simulink library "Encoders_Lib"  (R2023a)
settings: Solver=ode45  StartTime=0.0  StopTime=10.0  RelTol=1e-3  EnableMultiTasking=on
settings Model: Creator=uzivatel  LastModifiedBy=Jozko Mrkvicka
settings SolverCC: AlgebraicLoopSolver=TrustRegion
settings DataIOCC: LimitDataPoints=on  SaveFormat=Array  ReturnWorkspaceOutputs=off
settings OptimizationCC: LifeSpan=inf
settings DebuggingCC: UnderspecifiedInitializationDetection=Classic  MergeDetectMultiDrivingBlocksExec=none  SolverPrmCheckMsg=warning  UnconnectedInputMsg=warning  UnconnectedOutputMsg=warning  UnconnectedLineMsg=warning  StateNameClashWarn=warning  SFUnexpectedBacktrackingDiag=warning  SFNoUnconditionalDefaultTransitionDiag=warning  ArithmeticOperatorsInVariantConditions=warning
settings HardwareCC: ProdBitPerPointer=32  ProdBitPerSizeT=32  ProdBitPerPtrDiffT=32  ProdLargestAtomicFloat=None  ProdIntDivRoundTo=Undefined  ProdEndianess=Unspecified  ProdWordSize=32  ProdHWDeviceType=32-bit Generic
settings ModelReferenceCC: EnableRefExpFcnMdlSchedulingChecks=on  PropagateSignalLabelsOutOfModel=off
settings SFSimCC: SimUseLocalCustomCode=off  CustomCodeUndefinedFunction=UseInterfaceOnly
settings RTWCC: RTWUseLocalCustomCode=off
settings CodeAppCC: StateflowObjectComments=on
settings GRTTargetCC: TargetLangStandard=C89/C90 (ANSI)
settings ConfigComp: CovMetricSettings=dw  CovSaveCumulativeToWorkspaceVar=on  CovSaveSingleToWorkspaceVar=on  CovExternalEMLEnable=off

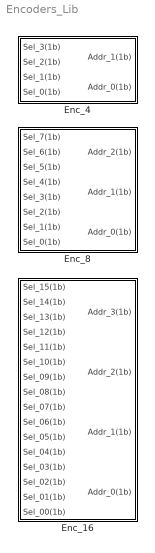
== system Encoders_Lib ==
  Enc_16 : Subsystem
  Enc_4 : Subsystem
  Enc_8 : Subsystem

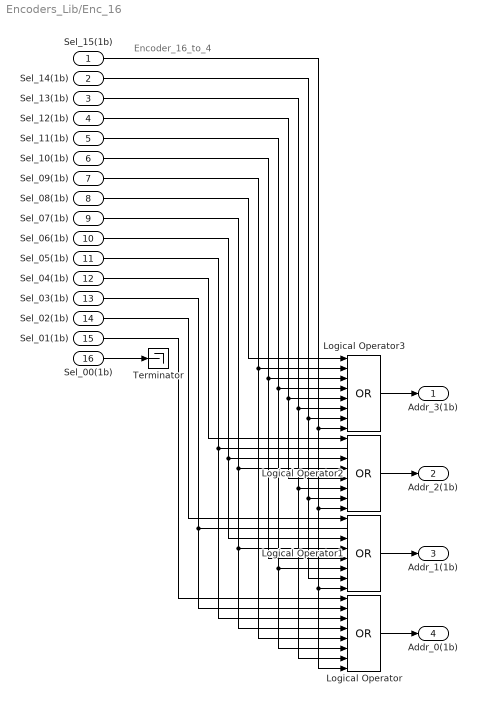
== system Encoders_Lib/Enc_16 ==
  note: Encoder_16_to_4
  Sel_15(1b) : Inport
  Sel_14(1b) : Inport  Port=2
  Sel_13(1b) : Inport  Port=3
  Sel_12(1b) : Inport  Port=4
  Sel_11(1b) : Inport  Port=5
  Sel_10(1b) : Inport  Port=6
  Sel_09(1b) : Inport  Port=7
  Sel_08(1b) : Inport  Port=8
  Sel_07(1b) : Inport  Port=9
  Sel_06(1b) : Inport  Port=10
  Sel_05(1b) : Inport  Port=11
  Sel_04(1b) : Inport  Port=12
  Sel_03(1b) : Inport  Port=13
  Sel_02(1b) : Inport  Port=14
  Sel_01(1b) : Inport  Port=15
  Sel_00(1b) : Inport  Port=16
  Logical Operator{,1..3} (4 alike) : Logic  Operator=OR  Inputs=8  IconShape=distinctive  AllPortsSameDT=off  OutDataTypeStr=boolean
  Terminator : Terminator
  Addr_3(1b) : Outport
  Addr_2(1b) : Outport  Port=2
  Addr_1(1b) : Outport  Port=3
  Addr_0(1b) : Outport  Port=4
  wires:
  Logical Operator/1 -> Addr_0(1b)/1
  Logical Operator1/1 -> Addr_1(1b)/1
  Logical Operator2/1 -> Addr_2(1b)/1
  Logical Operator3/1 -> Addr_3(1b)/1
  Sel_01(1b)/1 -> Logical Operator/1
  Sel_02(1b)/1 -> Logical Operator1/1
  Sel_03(1b)/1 -> Logical Operator1/2, Logical Operator/2
  Sel_04(1b)/1 -> Logical Operator2/1
  Sel_05(1b)/1 -> Logical Operator2/2, Logical Operator/3
  Sel_06(1b)/1 -> Logical Operator2/3, Logical Operator1/3
  Sel_07(1b)/1 -> Logical Operator2/4, Logical Operator/4, Logical Operator1/4
  Sel_08(1b)/1 -> Logical Operator3/1
  Sel_09(1b)/1 -> Logical Operator/5, Logical Operator3/2
  Sel_10(1b)/1 -> Logical Operator1/5, Logical Operator3/3
  Sel_11(1b)/1 -> Logical Operator3/4, Logical Operator/6, Logical Operator1/6
  Sel_12(1b)/1 -> Logical Operator2/5, Logical Operator3/5
  Sel_13(1b)/1 -> Logical Operator/7, Logical Operator2/6, Logical Operator3/6
  Sel_14(1b)/1 -> Logical Operator3/7, Logical Operator1/7, Logical Operator2/7
  Sel_15(1b)/1 -> Logical Operator/8, Logical Operator1/8, Logical Operator2/8, Logical Operator3/8
  Sel_00(1b)/1 -> Terminator/1

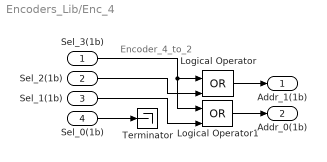
== system Encoders_Lib/Enc_4 ==
  note: Encoder_4_to_2
  Sel_3(1b) : Inport
  Sel_2(1b) : Inport  Port=2
  Sel_1(1b) : Inport  Port=3
  Sel_0(1b) : Inport  Port=4
  Logical Operator : Logic  Operator=OR  IconShape=distinctive  AllPortsSameDT=off  OutDataTypeStr=boolean
  Logical Operator1 : Logic  Operator=OR  IconShape=distinctive  AllPortsSameDT=off  OutDataTypeStr=boolean
  Terminator : Terminator
  Addr_1(1b) : Outport
  Addr_0(1b) : Outport  Port=2
  wires:
  Logical Operator/1 -> Addr_1(1b)/1
  Logical Operator1/1 -> Addr_0(1b)/1
  Sel_2(1b)/1 -> Logical Operator/2
  Sel_1(1b)/1 -> Logical Operator1/2
  Sel_0(1b)/1 -> Terminator/1
  Sel_3(1b)/1 -> Logical Operator/1, Logical Operator1/1

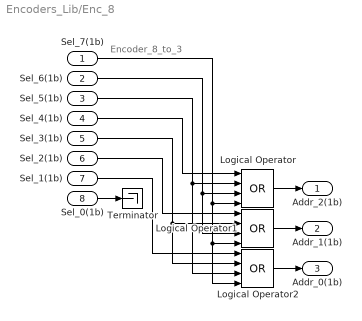
== system Encoders_Lib/Enc_8 ==
  note: Encoder_8_to_3
  Sel_7(1b) : Inport
  Sel_6(1b) : Inport  Port=2
  Sel_5(1b) : Inport  Port=3
  Sel_4(1b) : Inport  Port=4
  Sel_3(1b) : Inport  Port=5
  Sel_2(1b) : Inport  Port=6
  Sel_1(1b) : Inport  Port=7
  Sel_0(1b) : Inport  Port=8
  Logical Operator : Logic  Operator=OR  Inputs=4  IconShape=distinctive  AllPortsSameDT=off  OutDataTypeStr=boolean
  Logical Operator1 : Logic  Operator=OR  Inputs=4  IconShape=distinctive  AllPortsSameDT=off  OutDataTypeStr=boolean
  Logical Operator2 : Logic  Operator=OR  Inputs=4  IconShape=distinctive  AllPortsSameDT=off  OutDataTypeStr=boolean
  Terminator : Terminator
  Addr_2(1b) : Outport
  Addr_1(1b) : Outport  Port=2
  Addr_0(1b) : Outport  Port=3
  wires:
  Logical Operator/1 -> Addr_2(1b)/1
  Logical Operator1/1 -> Addr_1(1b)/1
  Logical Operator2/1 -> Addr_0(1b)/1
  Sel_4(1b)/1 -> Logical Operator/1
  Sel_2(1b)/1 -> Logical Operator1/1
  Sel_6(1b)/1 -> Logical Operator/3, Logical Operator1/3
  Sel_5(1b)/1 -> Logical Operator/2, Logical Operator2/3
  Sel_3(1b)/1 -> Logical Operator2/2, Logical Operator1/2
  Sel_7(1b)/1 -> Logical Operator/4, Logical Operator2/4, Logical Operator1/4
  Sel_0(1b)/1 -> Terminator/1
  Sel_1(1b)/1 -> Logical Operator2/1
